simulink model "SimuHybrid_Ex1"  (R2024a)
settings: Solver=FixedStepAuto  StartTime=ti  StopTime=tf  FixedStep=1e-3  MaxStep=1e-3  RelTol=1e-5  AbsTol=1e-8
settings Model: Creator=perruquetti  LastModifiedBy=perruquetti
settings SolverCC: AlgebraicLoopSolver=LineSearch
settings DebuggingCC: AlgebraicLoopMsg=none  UnconnectedInputMsg=warning  UnconnectedOutputMsg=warning  UnconnectedLineMsg=warning
settings ModelReferenceCC: EnableRefExpFcnMdlSchedulingChecks=on
settings RTWCC: GPUComputeCapability=3.5  DLArmComputeVersion=19.05

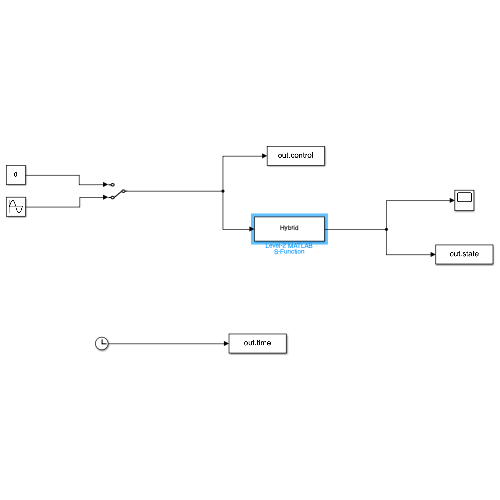
[thumbnail: Simulink's stored preview of the top-level diagram]
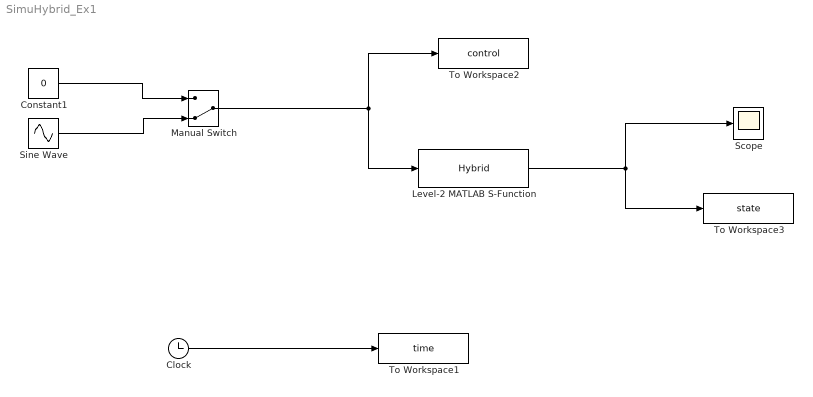
== system SimuHybrid_Ex1 ==
  Clock : Clock
  Constant1 : Constant  Value=0
  Level-2 MATLAB S-Function : M-S-Function  FunctionName=Hybrid
  Manual Switch : ManualSwitch  CurrentSetting=0
  Scope : Scope
  Sine Wave : Sin  SampleTime=0
  To Workspace1 : ToWorkspace  VariableName=time  SampleTime=-1
  To Workspace2 : ToWorkspace  VariableName=control  SampleTime=-1
  To Workspace3 : ToWorkspace  VariableName=state  SampleTime=-1
  wires:
  Clock/1 -> To Workspace1/1
  Level-2 MATLAB S-Function/1 -> Scope/1, To Workspace3/1
  Constant1/1 -> Manual Switch/1
  Sine Wave/1 -> Manual Switch/2
  Manual Switch/1 -> Level-2 MATLAB S-Function/1, To Workspace2/1
